simulink model "Drone_NAV_SLAM"  (R2024a)
settings: Solver=FixedStepAuto  StartTime=0.0  StopTime=inf  FixedStep=0.05  RelTol=1e-3
undefined symbols (not defined in the file): DiscIntNeverNeededParam
libraries: robotcorelib x5, mspfiltlib x1
settings Model: Creator=quentinlandon  LastModifiedBy=user
settings SolverCC: AllowMultiTaskInputOutput=on  ConcurrentTasks=on
settings SFSimCC: SimTargetLang=C++

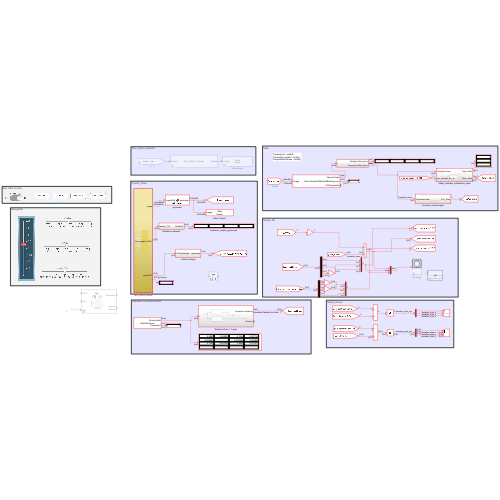
[thumbnail: Simulink's stored preview of the top-level diagram]
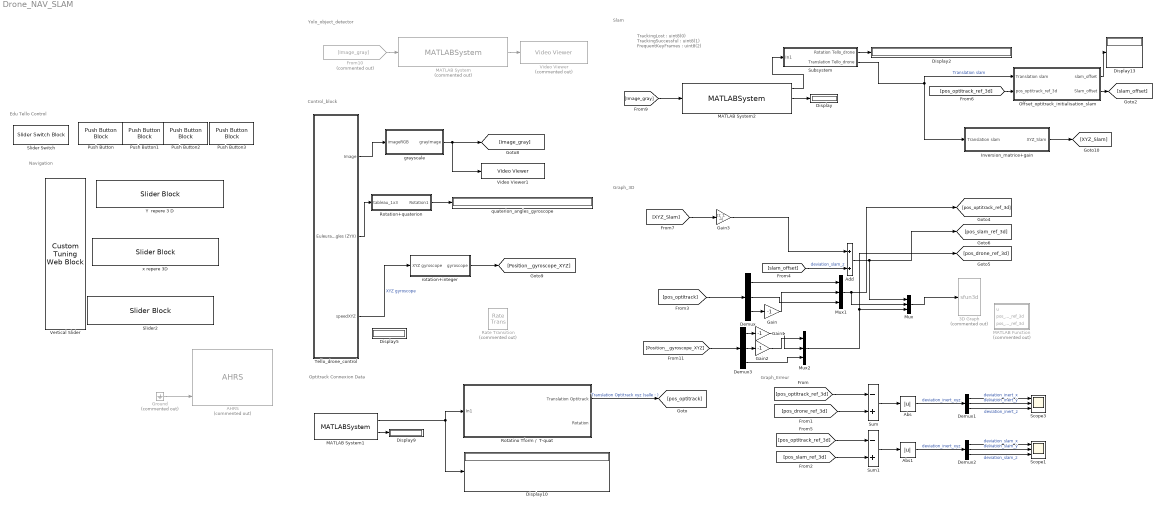
== system Drone_NAV_SLAM ==
  note: Control_block
  note: Graph_Erreur
  note: Graph_3D
  note: Slam
  note: Yolo_object_detector
  note: Optitrack Connexion Data
  note: TrackingLost : uint8(0)
      | TrackingSuccessful : uint8(1)
      | FrequentKeyFrames : uint8(2)
  note: Navigation
  note: Edu Tello Control
  3D Graph : S-Function  Commented=on  LoadFcn=if exist('sfun3d','file'), sfun3d([],[],[],'LoadBlock'); end  FunctionName=sfun3d  Parameters=ax,T,np,cp,gd,ls,mk,mx,hd,tb  SFunctionDeploymentMode=off  EnableBusSupport=off  mask(3D Graph){np=3, ax=[-5 5 -5 5 -5 5], mx=1e4, T=-1, cp=[3 2 1], gd=on, hd=off, tb=on, ls=-, mk=none}
      mask prompts: np "Number of moving points (lines)"; ax "Range: [xmin xmax  ymin ymax zmin zmax]"; mx "Max number of points in each line"; T "Sampling Time"; cp "Camera position (use [0 0 1] for 2D XY view)"; gd "Grid (on|off)"; hd "HeadMarkers (on|off)"; tb "Toolbar (on|off)"; ls "LineStyle"; mk "LineMarker"
      mask help:
      | This block plots the position of several points in the XYZ space. The input contains the coordinates of all the points (x1,y1,z1,x2,y2,z2,...).
      | The number of moving points (lines), the XYZ ranges, sampling time, camera position, and grid (among other things) can be set as mask parameters.
      settings: CopyFcn=if exist('sfun3d','file'), sfun3d([],[],[],'CopyBlock'); end  DeleteFcn=if exist('sfun3d','file'), sfun3d([],[],[],'DeleteBlock'); end  NameChangeFcn=if exist('sfun3d','file'), sfun3d([],[],[],'NameChange'); end
      mask Help:
      | This block plots the position of several points in the XYZ space. The input contains the coordinates of all the points (x1,y1,z1,x2,y2,z2,...).
      | The number of moving points (lines), the XYZ ranges, sampling time, camera position, and grid (among other things) can be set as mask parameters.
      mask TypeOptions ls: - | -- | : | -. | none
      mask TypeOptions mk: none | . | + | o | * | x | square | diamond | v | ^ | > | < | pentagram | hexagram
      mask Display: plot([.05 .95 .95 .05 .05],[.45 .45 .95 .95 .45], 0.5+cos(0:0.1:2*pi)*0.3,0.7+sin(0:0.1:2*pi)*0.2)
  AHRS : mspfiltlib/AHRS  Commented=on  DispRefFrame=NED  DecimationFactor=1  InitialProcessNoise=ahrsfilter.defaultProcessNoise  OrientationFormat=quaternion  SimulateUsing=Interpreted execution  AccelerometerNoise=0.0001924722  GyroscopeNoise=9.1385e-5  MagnetometerNoise=0.1  GyroscopeDriftNoise=3.0462e-13  LinearAccelerationNoise=0.0096236100000000012  MagneticDisturbanceNoise=0.5  LinearAccelerationDecayFactor=0.5  MagneticDisturbanceDecayFactor=0.5  ExpectedMagneticFieldStrength=50
  Abs : Abs  SaturateOnIntegerOverflow=off
  Abs1 : Abs  SaturateOnIntegerOverflow=off
  Add : Sum
  Demux{,1..3} (4 alike) : Demux  Outputs=3
  Display{,2,5,9..10,13} (6 alike) : Display
  From10 : From  Commented=on  GotoTag=Image_gray
  Gain : Gain  Gain=-1
  Gain1 : Gain  Gain=-1
  Gain2 : Gain  Gain=-1
  Gain3 : Gain  Gain=[1; 1; -1]
  Ground : Ground  Commented=on
  Inversion_matrice+gain : Subsystem
  MATLAB Function : MATLAB Function  Commented=on  TreatAsAtomicUnit=on
  MATLAB System : MATLABSystem  Commented=on  System=Yolo_Object_Detector  SimulateUsing=Interpreted execution
      mask Type: Yolo_Object_Detector
      mask Display:
      | disp('Yolo_Object_Detector');
      | port_label('input',1,'Image');
      | port_label('output',1,'Image');
  MATLAB System1 : MATLABSystem  System=OptilinkSystem  HostIP=127.0.0.1  ClientIP=127.0.0.1  SimulateUsing=Interpreted execution
      mask Type: OptilinkSystem
      mask Display:
      | disp('OptilinkSystem');
      | port_label('output',1,'Drones data');
      | port_label('output',2,'Connected');
  MATLAB System2 : MATLABSystem  System=MonoVisualSLAMSystem  FocalLength=[366.7411, 362.9497 ]  PrincipalPoint=[ 252.67, 206.61 ]  ImageSize=[ 360, 480 ]  SimulateUsing=Code generation
      mask Type: MonoVisualSLAMSystem
      mask Display:
      | disp('MonoVisualSLAMSystem');
      | port_label('input',1,'Image');
      | port_label('output',1,'Camera Pose');
      | port_label('output',2,'Tracking Lost');
      | port_label('output',3,'XYZmappoints');
  Mux : Mux  Inputs=3
  Mux1 : Mux  Inputs=3
  Mux2 : Mux  Inputs=3
  Offset_optitrack_initialisation_slam : Subsystem
  Push Button : PushButtonBlock  ButtonText=Takeoff  OffValue=0.000000
  Push Button1 : PushButtonBlock  ButtonText=Land  OffValue=0.000000
  Push Button2 : PushButtonBlock  ButtonText=MoveXYZ  OffValue=0.000000
  Push Button3 : PushButtonBlock  ButtonText=Moverotate  OffValue=0.000000
  Rate Transition : RateTransition  Commented=on
  Rotatino Tform /  T-quat : Subsystem
  Rotation+quaterion : Subsystem
  Scope1 : Scope  NumInputPorts=3
  Scope3 : Scope  NumInputPorts=3
  Slider Switch : SliderSwitchBlock
      settings: Values={{'Off', 'On'}, [0 1]}
  Slider2 : SliderBlock  ScaleMin=-180  ScaleMax=180
  Subsystem : Subsystem
  Sum : Sum  Inputs=-+
  Sum1 : Sum  Inputs=-+
  Tello_drone_control : Subsystem
  Vertical Slider : CustomTuningWebBlock  LabelPosition=Hide  ShowInitialText=on  Configuration="{\"components\":[{\"name\":\"LinearScaleComponent\",\"settings\":{\"bounds\":{\"max\":2,\"min\":-2,\"tickInterval\":\"auto\"},\"internalTickHeightScaleFactor\":0.5,\"labelColor\":[255,255,200],\"labelFont\":{\"font\":\"Arial\",\"fontSize\":12},\"labelOffset\":0.05,\"labelTransparency\":1,\"needleImage\":{\"size\":[596,842],\"src\":\"data:image\\/svg+xml;base64,PD94bWwgdmVyc2lvbj0iMS4wIiBlbmNvZGluZz0idXRmLTgiPz4NCjwhLS0gR2VuZXJhdG9yOiBBZG9iZSBJbGx1c3RyYXRvciAyNS4wLjAsIFNWRyBFeHBvcnQgUGx1Zy1JbiAuIFNWRyBWZXJzaW9uOiA2LjAwIEJ1aWxkIDApICAtLT4NCjxzdmcgdmVyc2lvbj0iMS4xIg0KCSBpZD0ic3ZnOCIgeG1sbnM6Y2M9Imh0dHA6Ly9jcmVhdGl2ZWNvbW1vbnMub3JnL25zIyIgeG1sbnM6ZGM9Imh0dHA6Ly9wdXJsLm9yZy9kYy9lbGVtZW50cy8xLjEvIiB4bWxuczppbmtzY2FwZT0iaHR0cDovL3d3dy5pbmtzY2FwZS5vcmcvbmFtZXNw ...(+2420 chars)\",\"srcOrientation\":\"horizontal\"},\"needleOffset\":[0.0642123287671233,-0.8044596912521441],\"needleSize\":{\"height\":0.07668067226890757,\"width\":0.4337797619047619},\"position\":[0.03623949579831933,0.2829861111111111,0.6088789682539683,0.9196428571428571],\"referencePoint\":\"auto\",\"scaleColors\":[],\"scaleColorsSize\":0.2,\"scaleDirection\":\"BT\",\"showLabels\":1,\"showMinorTicks\":0,\"showSpanLine\":1,\"showTicks\":1,\"tickColor\":[252,252,197],\"tickTransparency\":1,\"valueBarColor\":[0,114,189],\"valueBarOffset\":-0.27,\"valueBarSize\":0.1,\"valueBarTransparency\":1}},{\"name\":\"BackgroundImageComponent\",\"settings\":{\"image\":{\"size\":[380,101],\"src\":\"data:image\\/svg+xml;base64,PHN2ZyB4bWxucz0iaHR0cDovL3d3dy53My5vcmcvMjAwMC9zdmciIHhtbG5zOnhsaW5rPSJodHRwOi8vd3d3LnczLm9yZy8xOTk5L3hsaW5rIiB2aWV3Qm94PSIwIDAgMzgwIDEwMSI+PGRlZnM+PHN0eWxlPi5jbHMtMXtmaWxsOiMwMDJiNDI7fS5jbHMtMntmaWxsOiM0MjcwODI7fS5jbHMtM3tmaWxsOnVybCgjcmFkaWFsLWdyYWRpZW50KTt9LmNscy00e2ZpbGw6I2M4YzhjODtzdHJva2U6IzAwMDt9PC9zdHlsZT48cmFkaWFsR3JhZGllbnQgaWQ9InJhZGlhbC1ncmFkaWVudCIgY3g9IjE5MCIgY3k9IjUwLjUiIHI9IjI2OS4yMSIgZ3JhZGllbnRVbml0cz0idXNlclNwYWNlT25Vc2UiPjxzdG9wIG9mZnNldD0iMC4wMSIgc3RvcC1jb2xvcj0iIzNlNGY1OCIvPjxzdG9wIG9mZnNldD0iMC4wNiIgc3RvcC1jb2xvcj0iIzQ0NTc2MSIvPjxzdG9wIG9mZnNldD0iMC4xNSIgc3RvcC1jb2xvcj0iIzU1NmE3NiIvPjxzdG9wIG9mZnNldD0iMC4yNSIgc3RvcC1jb2xvcj0iIzZkODg5NSIvPjxzdG9wIG9mZnNldD0iMC4zOCIgc3RvcC1jb2xvcj0iIzhmYjJjMyIvPjxzdG9wIG9mZnNldD0iMC41MiIgc3RvcC1jb2xvcj0iI2I2ZTRmYSIvPjxzdG9wIG9mZnNldD0iMSIgc3RvcC1jb2xvcj0iIzE1NDY1NyIvPjwvcmFkaWFsR3JhZGllbnQ+PC9kZWZzPjxnIGlkPSJmcmFtZSI+PGcgaWQ9IkxheWVyXzIiIGRhdGEtbmFtZT0iTGF5ZXIgMiI+PGcgaWQ9IkxheWVyXzEtMiIgZGF0YS1uYW1lPSJMYXllciAxLTIiPjxyZWN0IGlkPSJyZWN0MTAzNiIgY2xhc3M9ImNscy0xIiB4PSIxMSIgeT0iMTEiIHdpZHRoPSIzNTgiIGhlaWdodD0iNzkiLz48cGF0aCBpZD0icGF0aDEwMzgiIGNsYXNzPSJjbHMtMiIgZD0iTTgsOFY5M0gzNzJWOFpNMzY5LDkwSDExVjExSDM2OVoiLz48cGF0aCBpZD0icGF0aDEwNDAiIGNsYXNzPSJjbHMtMyIgZD0iTTAsMFYxMDFIMzgwVjBaTTM3Miw5M0g4VjhIMzcyWiIvPjwvZz48L2c+PC9nPjxnIGlkPSJ0cmFjayI+PHBhdGggaWQ9InJlY3QxNjExIiBjbGFzcz0iY2xzLTQiIGQ9Ik0zMy4zNywyNi41OUgzNDYuNjNjNCwwLDcuMjUsMi42LDcuMjUsNS44MWgwYzAsMy4yMS0zLjI1LDUuODItNy4yNSw1LjgySDMzLjM3Yy00LDAtNy4yNS0yLjYxLTcuMjUtNS44MmgwQzI2LjEyLDI5LjE5LDI5LjM3LDI2LjU5LDMzLjM3LDI2LjU5WiIvPjwvZz48L3N2Zz4=\",\"srcOrientation\":\"horizontal\"},\"position\":[0,0,1,1],\"scaleMode\":\"0\"}},{\"name\":\"ForegroundImageComponent\",\"settings\":{\"image\":{\"size\":[0,0],\"src\":\"default\",\"srcOrientation\":[]},\"isForeground\":1,\"position\":[0,0,1,1],\"scaleMode\":\"0\"}}],\"settings\":{\"BindingType\":\"param\",\"aspectRatio\":3.7777777777777777,\"backgroundColor\":[0,0,0,\"1\"],\"backgroundOffset\":0,\"backgroundOpacity\":1,\"fixedAspectRatio\":\"on\",\"foregroundColor\":[252,252,196],\"orientation\":\"vertical\",\"showBackgroundColor\":false,\"value\":0,\"version\":\"R2023a\"},\"type\":\"LinearGauge\"}"
  Video Viewer : VideoViewer  Commented=on  FigPos=[-468 812 418 304]
  Video Viewer1 : VideoViewer  FigPos=[-1122 1013 902 426]
  Y  repere 3 D : SliderBlock  ScaleMin=-2  ScaleMax=2
  grayscale : MATLAB Function  TreatAsAtomicUnit=on
  quaterion_angles_gyroscope : Display
  rotation+integer : Subsystem
  x repere 3D : SliderBlock  ScaleMin=-2  ScaleMax=2
  wires:
  MATLAB System2/2 -> Display/1
  Subsystem/1(Rotation Tello_drone) -> Display2/1
  ? -> Display5/1
  MATLAB System1/2 -> Display9/1
  MATLAB System1/1 -> Rotatino Tform /  T-quat/1(In1), Display10/1
  Subsystem/2(Translation Tello_drone) -> Inversion_matrice+gain/1(Translation slam), Offset_optitrack_initialisation_slam/1(Translation slam)  "Translation slam"
  Tello_drone_control/3(speedXYZ) -> rotation+integer/1(XYZ gyroscope)  "XYZ gyroscope"
  Rotatino Tform /  T-quat/1(Translation Optitrack) -> [pos_optitrack]  "Translation Optitrack xyz (salle : )"
  [pos_optitrack_ref_3d] -> Sum/1
  [pos_drone_ref_3d] -> Sum/2
  Demux1/1 -> Scope3/1  "deviation_inert_x"
  Demux1/2 -> Scope3/2  "deviation_inert_y"
  Demux1/3 -> Scope3/3  "deviation_inert_z"
  Abs/1 -> Demux1/1  "deviation_inert_xyz"
  [pos_slam_ref_3d] -> Sum1/2
  Tello_drone_control/2(Euleurangles (ZYX)) -> Rotation+quaterion/1(tableau_1x3)
  Rotation+quaterion/1(Rotation1) -> quaterion_angles_gyroscope/1
  grayscale/1(grayImage) -> Video Viewer1/1, [Image_gray]
  Tello_drone_control/1(Image) -> grayscale/1(imageRGB)
  From10/1 -> MATLAB System/1
  MATLAB System/1 -> Video Viewer/1
  rotation+integer/1(gyroscope) -> [Position__gyroscope_XYZ]
  Offset_optitrack_initialisation_slam/1(slam_offset) -> Display13/1
  Inversion_matrice+gain/1(XYZ_Slam) -> [XYZ_Slam]
  Offset_optitrack_initialisation_slam/2(Slam_offset) -> [slam_offset]
  [pos_optitrack_ref_3d] -> Offset_optitrack_initialisation_slam/2(pos_optitrack_ref_3d)
  [slam_offset] -> Add/2  "deviation_slam_z"
  Mux/1 -> 3D Graph/1
  [Image_gray] -> MATLAB System2/1
  MATLAB System2/1 -> Subsystem/1(In1)
  Ground/1 -> AHRS/3
  Sum/1 -> Abs/1
  Abs1/1 -> Demux2/1  "deviation_inert_xyz"
  Sum1/1 -> Abs1/1
  Demux2/3 -> Scope1/3  "deviation_slam_z"
  Demux2/2 -> Scope1/2  "deviation_slam_y"
  Demux2/1 -> Scope1/1  "deviation_slam_x"
  [pos_optitrack_ref_3d] -> Sum1/1
  Gain/1 -> Mux1/2
  Demux/1 -> Mux1/1
  Demux/2 -> Mux1/3
  Demux/3 -> Gain/1
  [pos_optitrack] -> Demux/1
  Mux1/1 -> Mux/2, [pos_optitrack_ref_3d]
  Demux3/1 -> Gain1/1
  Gain1/1 -> Mux2/2
  Demux3/2 -> Gain2/1
  Gain2/1 -> Mux2/1
  Demux3/3 -> Mux2/3
  [Position__gyroscope_XYZ] -> Demux3/1
  Mux2/1 -> Mux/3, [pos_drone_ref_3d]
  [XYZ_Slam] -> Gain3/1
  Gain3/1 -> Add/1
  Add/1 -> Mux/1, [pos_slam_ref_3d]

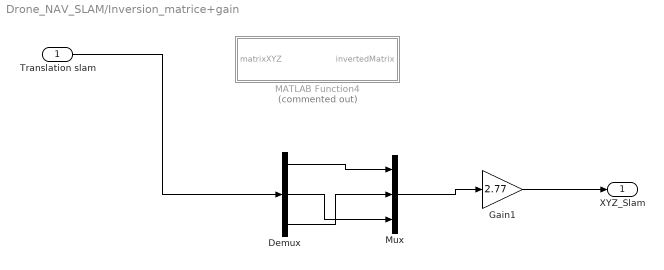
== system Drone_NAV_SLAM/Inversion_matrice+gain ==
  Translation slam : Inport
  Demux : Demux  Outputs=3
  Gain1 : Gain  Gain=2.77
  MATLAB Function4 : MATLAB Function  Commented=on  TreatAsAtomicUnit=on
  Mux : Mux  Inputs=3
  XYZ_Slam : Outport
  wires:
  Translation slam/1 -> Demux/1
  Gain1/1 -> XYZ_Slam/1
  Demux/1 -> Mux/1
  Demux/3 -> Mux/2
  Demux/2 -> Mux/3
  Mux/1 -> Gain1/1

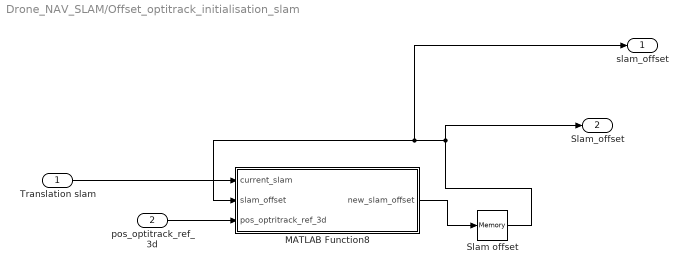
== system Drone_NAV_SLAM/Offset_optitrack_initialisation_slam ==
  Translation slam : Inport
  pos_optitrack_ref_3d : Inport  Port=2
  MATLAB Function8 : MATLAB Function  TreatAsAtomicUnit=on
  Slam offset : Memory  InitialCondition=[0;0;0]
  slam_offset : Outport
  Slam_offset : Outport  Port=2
  wires:
  MATLAB Function8/1(new_slam_offset) -> Slam offset/1
  Slam offset/1 -> Slam_offset/1, slam_offset/1, MATLAB Function8/2(slam_offset)
  Translation slam/1 -> MATLAB Function8/1(current_slam)
  pos_optitrack_ref_3d/1 -> MATLAB Function8/3(pos_optritrack_ref_3d)

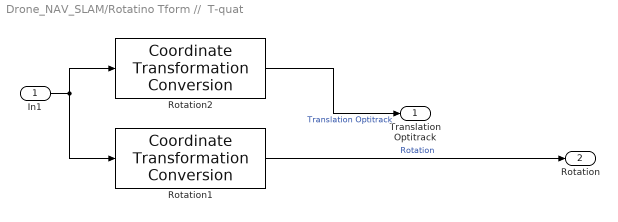
== system Drone_NAV_SLAM/Rotatino Tform //  T-quat ==
  In1 : Inport
  Rotation1 : robotcorelib/Coordinate Transformation Conversion  InputRepresentation=Homogeneous Transformation  InputEulerSequence=ZYX  ShowTrVecInputPort=on  OutputRepresentation=Quaternion  OutputEulerSequence=ZYX  ShowTrVecOutputPort=off  SimulateUsing=Code generation
      settings: LibrarySourceBlock=uavutilslib/Coordinate Transformation Conversion
  Rotation2 : robotcorelib/Coordinate Transformation Conversion  InputRepresentation=Homogeneous Transformation  InputEulerSequence=ZYX  ShowTrVecInputPort=on  OutputRepresentation=Translation Vector  OutputEulerSequence=ZYX  ShowTrVecOutputPort=off  SimulateUsing=Code generation
      settings: LibrarySourceBlock=uavutilslib/Coordinate Transformation Conversion
  Translation Optitrack : Outport
  Rotation : Outport  Port=2
  wires:
  Rotation1/1 -> Rotation/1  "Rotation"
  Rotation2/1 -> Translation Optitrack/1  "Translation Optitrack"
  In1/1 -> Rotation2/1, Rotation1/1

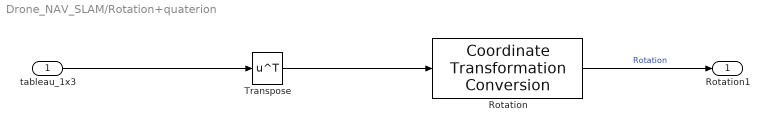
== system Drone_NAV_SLAM/Rotation+quaterion ==
  tableau_1x3 : Inport
  Rotation : robotcorelib/Coordinate Transformation Conversion  InputRepresentation=Euler Angles  InputEulerSequence=ZYX  ShowTrVecInputPort=on  OutputRepresentation=Quaternion  OutputEulerSequence=ZYX  ShowTrVecOutputPort=off  SimulateUsing=Code generation
      settings: LibrarySourceBlock=uavutilslib/Coordinate Transformation Conversion
  Transpose : Math  Operator=transpose
  Rotation1 : Outport
  wires:
  Rotation/1 -> Rotation1/1  "Rotation"
  Transpose/1 -> Rotation/1
  tableau_1x3/1 -> Transpose/1

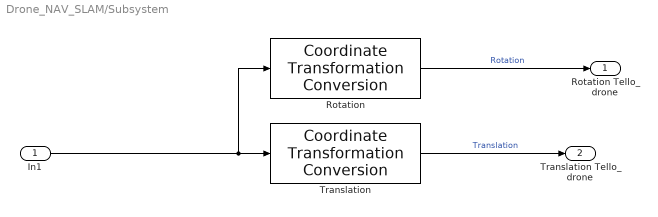
== system Drone_NAV_SLAM/Subsystem ==
  In1 : Inport
  Rotation : robotcorelib/Coordinate Transformation Conversion  InputRepresentation=Homogeneous Transformation  InputEulerSequence=ZYX  ShowTrVecInputPort=on  OutputRepresentation=Quaternion  OutputEulerSequence=ZYX  ShowTrVecOutputPort=off  SimulateUsing=Code generation
      settings: LibrarySourceBlock=uavutilslib/Coordinate Transformation Conversion
  Translation : robotcorelib/Coordinate Transformation Conversion  InputRepresentation=Homogeneous Transformation  InputEulerSequence=ZYX  ShowTrVecInputPort=on  OutputRepresentation=Translation Vector  OutputEulerSequence=ZYX  ShowTrVecOutputPort=on  SimulateUsing=Code generation
      settings: LibrarySourceBlock=uavutilslib/Coordinate Transformation Conversion
  Rotation Tello_drone : Outport
  Translation Tello_drone : Outport  Port=2
  wires:
  Translation/1 -> Translation Tello_drone/1  "Translation"
  Rotation/1 -> Rotation Tello_drone/1  "Rotation"
  In1/1 -> Rotation/1, Translation/1

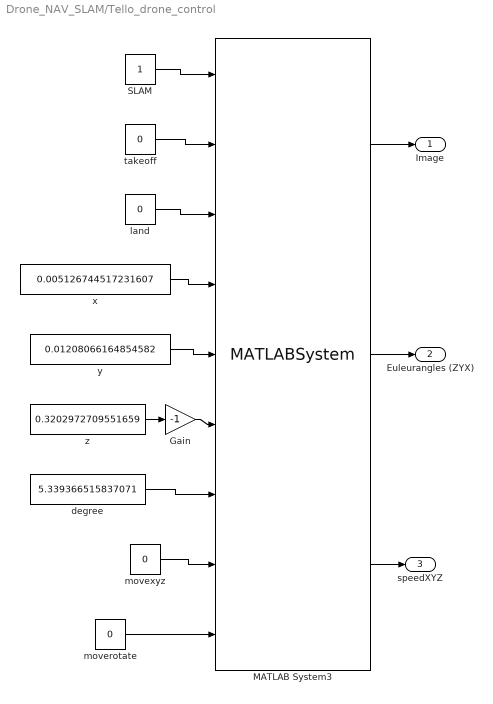
== system Drone_NAV_SLAM/Tello_drone_control ==
  Gain : Gain  Gain=-1
  MATLAB System3 : MATLABSystem  System=Tello_drone_control  droneIP=193.169.0.11  SimulateUsing=Interpreted execution
      mask Type: Tello_drone_control
      mask Display:
      | disp('Tello_drone_control');
      | port_label('input',1,'Slam');
      | port_label('input',2,'tkoff');
      | port_label('input',3,'landing');
      | port_label('input',4,'xMove');
      | port_label('input',5,'yMove');
      | port_label('input',6,'zMove');
      | port_label('input',7,'degree');
      | port_label('input',8,'movexyz');
      | port_label('input',9,'moverotate');
      | port_label('output',1,'imgresize');
      | port_label('output',2,'Eulerangles');
      | port_label('output',3,'speedXYZ');
  SLAM : Constant
  degree : Constant  Value=5.339366515837071
  land : Constant  Value=0
  moverotate : Constant  Value=0
  movexyz : Constant  Value=0
  takeoff : Constant  Value=0
  x : Constant  Value=0.005126744517231607
  y : Constant  Value=0.01208066164854582
  z : Constant  Value=0.3202972709551659
  Image : Outport
  Euleurangles (ZYX) : Outport  Port=2
  speedXYZ : Outport  Port=3
  wires:
  moverotate/1 -> MATLAB System3/9
  land/1 -> MATLAB System3/3
  y/1 -> MATLAB System3/5
  x/1 -> MATLAB System3/4
  Gain/1 -> MATLAB System3/6
  z/1 -> Gain/1
  degree/1 -> MATLAB System3/7
  SLAM/1 -> MATLAB System3/1
  movexyz/1 -> MATLAB System3/8
  MATLAB System3/1 -> Image/1
  takeoff/1 -> MATLAB System3/2
  MATLAB System3/2 -> Euleurangles (ZYX)/1
  MATLAB System3/3 -> speedXYZ/1

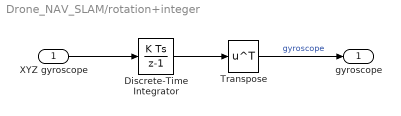
== system Drone_NAV_SLAM/rotation+integer ==
  XYZ gyroscope : Inport
  Discrete-Time Integrator : DiscreteIntegrator  SampleTime=-1  ICPrevOutput=DiscIntNeverNeededParam  ICPrevScaledInput=DiscIntNeverNeededParam
  Transpose : Math  Operator=transpose
  gyroscope : Outport
  wires:
  XYZ gyroscope/1 -> Discrete-Time Integrator/1
  Transpose/1 -> gyroscope/1  "gyroscope"
  Discrete-Time Integrator/1 -> Transpose/1

== matlab function Drone_NAV_SLAM/Inversion_matrice+gain/MATLAB Function4 ==
  data: matrixXYZ input; invertedMatrix output
function invertedMatrix = invertMatrix(matrixXYZ)    
    % Inverser la matrice
    invertedMatrix = [matrixXYZ(1); matrixXYZ(3); matrixXYZ(2)];
end

== matlab function Drone_NAV_SLAM/Offset_optitrack_initialisation_slam/MATLAB Function8 ==
  data: current_slam input; new_slam_offset output; slam_offset input; pos_optritrack_ref_3d input
function new_slam_offset = fcn(current_slam,slam_offset, pos_optritrack_ref_3d)

% If the slam started, and the Offset has not been set yet, assign the
% current Optitrack position 
if (any(current_slam) && ~any(slam_offset))
    new_slam_offset = pos_optritrack_ref_3d;
else
    new_slam_offset = slam_offset;
end 


%new_slam_offset(3) = 0;

== matlab function Drone_NAV_SLAM/MATLAB Function ==
  data: u input; pos_optitrack_ref_3d input; pos_drone_ref_3d input
function fcn(u, pos_optitrack_ref_3d, pos_drone_ref_3d)
% figure
hold on
plot3(u(1),u(2),u(3));

plot3(pos_optitrack_ref_3d(1),pos_optitrack_ref_3d(2),pos_optitrack_ref_3d(3));
plot3(pos_optitrack_ref_3d(1),pos_drone_ref_3d(2),pos_drone_ref_3d(3));

== matlab function Drone_NAV_SLAM/grayscale ==
  data: imageRGB input; grayImage output
function grayImage = rgbToGray(imageRGB)
    grayImage = rgb2gray(imageRGB);
end
